simulink model "W2P1_model"  (R2020a)
settings: Solver=FixedStepDiscrete  StartTime=0.0  StopTime=20  FixedStep=1  RelTol=1e-3
settings Model: Creator=avn19  LastModifiedBy=avn19

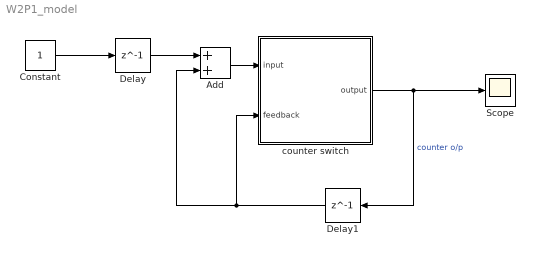
== system W2P1_model ==
  Add : Sum
  Constant : Constant
  Delay : Delay  DelayLength=1  InitialCondition=0
  Delay1 : Delay  DelayLength=1
  Scope : Scope
  counter switch : Stateflow chart  TreatAsAtomicUnit=on
  wires:
  Constant/1 -> Delay/1
  Delay/1 -> Add/1
  Add/1 -> counter switch/1(input)
  Delay1/1 -> counter switch/2(feedback), Add/2
  counter switch/1(output) -> Delay1/1, Scope/1  "counter o/p"

== stateflow chart W2P1_model/counter switch ==
  (default) -> (junction 48) : % switch
  (junction 48) -> (junction 49) [order 1] : [feedback >= 5]
  (junction 48) -> (junction 50) [order 2] : {output = input;}
  (junction 49) -> (junction 51) : {output = 0;}
  (junction 51) -> (junction 50)
  (junction 50) -> (junction 52)
  data: input input; output output; feedback input
